simulink model "scara_host"  (Simulink 8.1)
settings: Solver=FixedStepDiscrete  StartTime=0.0  StopTime=inf  RelTol=1e-3
libraries: simulink x7
settings Model: Creator=Sr Antonio  LastModifiedBy=sp
settings DebuggingCC: FcnCallInpInsideContextMsg=EnableAllAsWarning

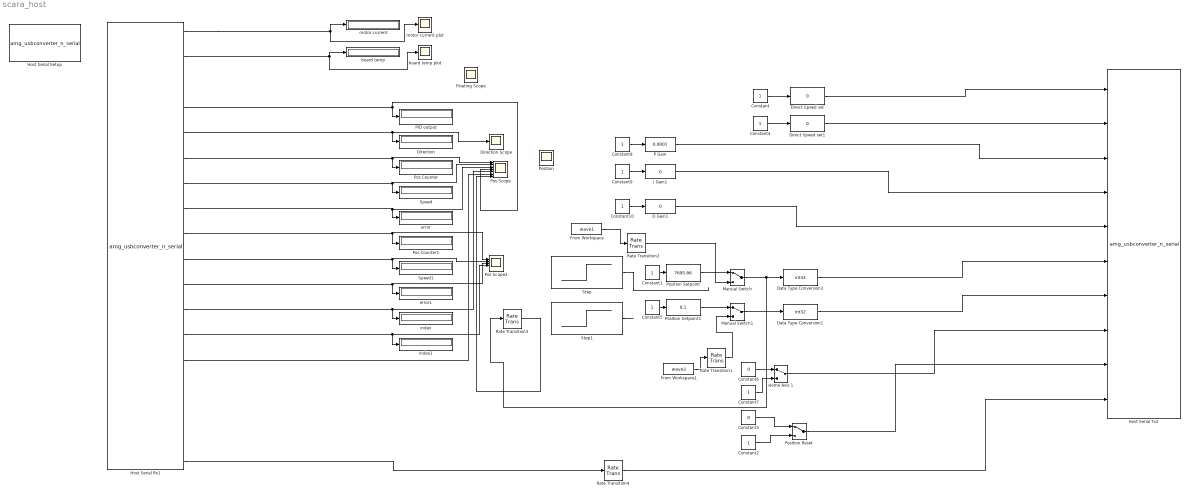
== system scara_host ==
  Constant{,4,8..10} (5 alike) : Constant
  Constant{1..2,5,7} (4 alike) : Constant  OutDataTypeStr=int32
  Constant3 : Constant  Value=0  OutDataTypeStr=int32
  Constant6 : Constant  Value=0  OutDataTypeStr=int32
  D Gain1 : simulink/Math Operations/Slider Gain  low=0  gain=0  high=10000
  Data Type Conversion1 : DataTypeConversion  OutDataTypeStr=int32
  Data Type Conversion3 : DataTypeConversion  OutDataTypeStr=int32
  Direct Speed set : simulink/Math Operations/Slider Gain  low=-1  gain=0  high=1
  Direct Speed set1 : simulink/Math Operations/Slider Gain  low=-1  gain=0  high=1
  Direction : Display
  Direction Scope : Scope
      settings: YMin=3e+07  YMax=3.35e+07  SaveName=ScopeData3
  Floating Scope : Scope
      settings: Floating=on  YMin=-12000  YMax=1000  SaveName=ScopeData5
  From Workspace : FromWorkspace  VariableName=wave1  SampleTime=0.001  Interpolate=off  OutputAfterFinalValue=Cyclic repetition
  From Workspace1 : FromWorkspace  VariableName=wave2  SampleTime=0.01  Interpolate=off  OutputAfterFinalValue=Cyclic repetition
  Home Axis 1 : ManualSwitch
  Host Serial Rx1 : S-Function  Priority=1  FunctionName=amg_usbconverter_n_serial  Parameters=configuration,port,transfer,baudrate,stopbit,inputtype,outputtype,binheaderarray,binterminatorarray,asciiheader,asciiterminator,bindatalength,packetmode,timeout,sampletime,sampletimestr,blockid  EnableBusSupport=off  mask(amg_usbconverter_n_serial){configuration=Rx, port=COM6, baudrate=115200, databits=8, parity=None, stopbit=1, flowcontrol=None, advanceoptions=off, rxbuffersize=2048, txbuffersize=2048, transfer=Blocking, timeout=2, packetmode=Binary, binheader='0E 0E', binterminator='0A 0A', porttype_double=4, porttype_single=0, porttype_int8=0, porttype_uint8=0, porttype_int16=0, porttype_uint16=0, porttype_int32=14, porttype_uint32=0, asciiformat='%d,%f', rx_asciiterminator=LF (0x0A - "\n"), tx_asciiterminator=LF (0x0A - "\n"), inputtype=[0], outputtype=[18  0 0 0 0 6 6 6 6 6 6 6 6 6 6 6 6 6 6], binheaderarray=[2 14  14], binterminatorarray=[2 10  10], bindatalength=88, asciiheader=['%d,%f' uint8(10)], asciiterminator=[1 10], sampletime=0.001, sampletimestr=, blockid=HostSerialRx1}
      mask prompts: baudrate "Baud rate (bps)"; databits "Data bits"; stopbit "Stop bit"; flowcontrol "Hardware flow control"; advanceoptions "Advance options"; rxbuffersize "Rx buffer size (bytes)"; txbuffersize "Tx buffer size (bytes)"; timeout "Wait time-out (Seconds)"; packetmode "Packet mode"; binheader "Binary header (example: '7E 7E')"; binterminator "Binary terminator (example: '03 03')"; porttype_double "Number of data port, type DOUBLE"; porttype_single "Number of data port, type SINGLE"; porttype_int8 "Number of data port, type INT8"; porttype_uint8 "Number of data port, type UINT8"; porttype_int16 "Number of data port, type INT16"; porttype_uint16 "Number of data port, type UINT16"; porttype_int32 "Number of data port, type INT32"; porttype_uint32 "Number of data port, type UINT32"; asciiformat "Ascii format"; rx_asciiterminator "End of packet"; tx_asciiterminator "End of packet"; inputtype "Input data type"; outputtype "Output data type"; binheaderarray "Binary header"; binterminatorarray "Binary terminator"; bindatalength "Binary data length"; asciiheader "Ascii header (printf format)"; asciiterminator "Ascii terminator"; sampletime "Sample time (sec)"; sampletimestr "Compiled sample time (sec) in string"
      mask init:
      | amg_usbconverter_n_serial_callback('init');
      mask Help: web(fullfile(waijungdocroot,'amg_usbconverter_n_uart.htm'), '-browser')
      mask TypeOptions configuration: Setup | Tx | Rx
      mask Callback configuration: amg_usbconverter_n_serial_callback('configuration');
      mask TypeOptions port: COM6
      mask Callback port: amg_usbconverter_n_serial_callback('port');
      mask Callback baudrate: amg_usbconverter_n_serial_callback('baudrate');
      mask TypeOptions databits: 8
      mask TypeOptions parity: None
      mask TypeOptions stopbit: 1 | 1.5 | 2
      mask TypeOptions flowcontrol: None | RTS | CTS | RTS/CTS
      mask Callback flowcontrol: amg_usbconverter_n_serial_callback('flowcontrol');
      mask Callback advanceoptions: amg_usbconverter_n_serial_callback('advanceoptions');
      mask TypeOptions rxbuffersize: 16 | 32 | 64 | 128 | 256 | 512 | 1024 | 2048
      mask TypeOptions txbuffersize: 16 | 32 | 64 | 128 | 256 | 512 | 1024 | 2048
      mask TypeOptions transfer: Blocking | Non-Blocking
      mask Callback transfer: amg_usbconverter_n_serial_callback('transfer');
      mask TypeOptions packetmode: Ascii | Binary
      mask Callback packetmode: amg_usbconverter_n_serial_callback('packetmode');
      mask Callback binheader: amg_usbconverter_n_serial_callback('binheader');
      mask Callback binterminator: amg_usbconverter_n_serial_callback('binterminator');
      mask Callback porttype_double: amg_usbconverter_n_serial_callback('porttype');
      mask Callback porttype_single: amg_usbconverter_n_serial_callback('porttype');
      mask Callback porttype_int8: amg_usbconverter_n_serial_callback('porttype');
      mask Callback porttype_uint8: amg_usbconverter_n_serial_callback('porttype');
      mask Callback porttype_int16: amg_usbconverter_n_serial_callback('porttype');
      mask Callback porttype_uint16: amg_usbconverter_n_serial_callback('porttype');
      mask Callback porttype_int32: amg_usbconverter_n_serial_callback('porttype');
      mask Callback porttype_uint32: amg_usbconverter_n_serial_callback('porttype');
      mask Callback asciiformat: amg_usbconverter_n_serial_callback('asciiformat');
      mask TypeOptions rx_asciiterminator: CR (0x0D - "\r") | LF (0x0A - "\n") | CRLF (0x0D 0x0A - "\r\n")
      mask Callback rx_asciiterminator: amg_usbconverter_n_serial_callback('rx_asciiterminator');
      mask TypeOptions tx_asciiterminator: CR (0x0D - "\r") | LF (0x0A - "\n") | CRLF (0x0D 0x0A - "\r\n") | None
      mask Callback tx_asciiterminator: amg_usbconverter_n_serial_callback('tx_asciiterminator');
      mask Callback sampletime: amg_usbconverter_n_serial_callback('sampletime');
      mask Callback sampletimestr: amg_usbconverter_n_serial_callback('sampletimestr');
      mask Callback blockid: amg_usbconverter_n_serial_callback('blockid');
      mask Display: text(0.05, 0.5, 'Obsolete !!!\nPort: COM6\nPacket: Binary\nTransfer: Blocking\nTs (sec): 0.001','ver','middle','hor','left');port_label('output', 1,'double');port_label('output', 2,'double');port_label('output', 3,'double');port_label('output', 4,'double');port_label('output', 5,'int32');port_label('output', 6,'int32');port_label('output', 7,'int32');port_label('output', 8,'int32');port_label('output', 9,'int32');port_label('output', 10,'int32');port_label('output', 11,'int32');port_label('output', 12,'int32');port_label('output', 13,'int32');port_label('output', 14,'int32');port_label('output', 15,'int32');port_label('output', 16,'int32');port_label('output', 17,'int32');port_label('output', 18,'int32');
  Host Serial Setup : S-Function  Priority=1  FunctionName=amg_usbconverter_n_serial  Parameters=configuration,port,transfer,baudrate,stopbit,inputtype,outputtype,binheaderarray,binterminatorarray,asciiheader,asciiterminator,bindatalength,packetmode,timeout,sampletime,sampletimestr,blockid  EnableBusSupport=off  mask(amg_usbconverter_n_serial){configuration=Setup, port=COM6, baudrate=10000000, databits=8, parity=None, stopbit=1, flowcontrol=None, advanceoptions=off, rxbuffersize=2048, txbuffersize=2048, transfer=Blocking, timeout=5, packetmode=Binary, binheader='7E 7E', binterminator='03 03', porttype_double=1, porttype_single=0, porttype_int8=1, porttype_uint8=0, porttype_int16=0, porttype_uint16=0, porttype_int32=0, porttype_uint32=0, asciiformat='%d,%f', rx_asciiterminator=CRLF (0x0D 0x0A - "\r\n"), tx_asciiterminator=CR (0x0D - "\r"), inputtype=[0], outputtype=[0], binheaderarray=[2 126  126], binterminatorarray=[2 3  3], bindatalength=0, asciiheader='', asciiterminator=[0], sampletime=inf, sampletimestr=, blockid=HostSerialSetup}
      mask prompts: baudrate "Baud rate (bps)"; databits "Data bits"; stopbit "Stop bit"; flowcontrol "Hardware flow control"; advanceoptions "Advance options"; rxbuffersize "Rx buffer size (bytes)"; txbuffersize "Tx buffer size (bytes)"; timeout "Wait time-out (Seconds)"; packetmode "Packet mode"; binheader "Binary header (example: '7E 7E')"; binterminator "Binary terminator (example: '03 03')"; porttype_double "Number of data port, type DOUBLE"; porttype_single "Number of data port, type SINGLE"; porttype_int8 "Number of data port, type INT8"; porttype_uint8 "Number of data port, type UINT8"; porttype_int16 "Number of data port, type INT16"; porttype_uint16 "Number of data port, type UINT16"; porttype_int32 "Number of data port, type INT32"; porttype_uint32 "Number of data port, type UINT32"; asciiformat "Ascii format"; rx_asciiterminator "End of packet"; tx_asciiterminator "End of packet"; inputtype "Input data type"; outputtype "Output data type"; binheaderarray "Binary header"; binterminatorarray "Binary terminator"; bindatalength "Binary data length"; asciiheader "Ascii header (printf format)"; asciiterminator "Ascii terminator"; sampletime "Sample time (sec)"; sampletimestr "Compiled sample time (sec) in string"
      mask init:
      | amg_usbconverter_n_serial_callback('init');
      mask Help: web(fullfile(waijungdocroot,'amg_usbconverter_n_uart.htm'), '-browser')
      mask TypeOptions configuration: Setup | Tx | Rx
      mask Callback configuration: amg_usbconverter_n_serial_callback('configuration');
      mask TypeOptions port: COM6
      mask Callback port: amg_usbconverter_n_serial_callback('port');
      mask Callback baudrate: amg_usbconverter_n_serial_callback('baudrate');
      mask TypeOptions databits: 8
      mask TypeOptions parity: None
      mask TypeOptions stopbit: 1 | 1.5 | 2
      mask TypeOptions flowcontrol: None | RTS | CTS | RTS/CTS
      mask Callback flowcontrol: amg_usbconverter_n_serial_callback('flowcontrol');
      mask Callback advanceoptions: amg_usbconverter_n_serial_callback('advanceoptions');
      mask TypeOptions rxbuffersize: 16 | 32 | 64 | 128 | 256 | 512 | 1024 | 2048
      mask TypeOptions txbuffersize: 16 | 32 | 64 | 128 | 256 | 512 | 1024 | 2048
      mask TypeOptions transfer: Blocking | Non-Blocking
      mask Callback transfer: amg_usbconverter_n_serial_callback('transfer');
      mask TypeOptions packetmode: Ascii | Binary
      mask Callback packetmode: amg_usbconverter_n_serial_callback('packetmode');
      mask Callback binheader: amg_usbconverter_n_serial_callback('binheader');
      mask Callback binterminator: amg_usbconverter_n_serial_callback('binterminator');
      mask Callback porttype_double: amg_usbconverter_n_serial_callback('porttype');
      mask Callback porttype_single: amg_usbconverter_n_serial_callback('porttype');
      mask Callback porttype_int8: amg_usbconverter_n_serial_callback('porttype');
      mask Callback porttype_uint8: amg_usbconverter_n_serial_callback('porttype');
      mask Callback porttype_int16: amg_usbconverter_n_serial_callback('porttype');
      mask Callback porttype_uint16: amg_usbconverter_n_serial_callback('porttype');
      mask Callback porttype_int32: amg_usbconverter_n_serial_callback('porttype');
      mask Callback porttype_uint32: amg_usbconverter_n_serial_callback('porttype');
      mask Callback asciiformat: amg_usbconverter_n_serial_callback('asciiformat');
      mask TypeOptions rx_asciiterminator: CR (0x0D - "\r") | LF (0x0A - "\n") | CRLF (0x0D 0x0A - "\r\n")
      mask Callback rx_asciiterminator: amg_usbconverter_n_serial_callback('rx_asciiterminator');
      mask TypeOptions tx_asciiterminator: CR (0x0D - "\r") | LF (0x0A - "\n") | CRLF (0x0D 0x0A - "\r\n") | None
      mask Callback tx_asciiterminator: amg_usbconverter_n_serial_callback('tx_asciiterminator');
      mask Callback sampletime: amg_usbconverter_n_serial_callback('sampletime');
      mask Callback sampletimestr: amg_usbconverter_n_serial_callback('sampletimestr');
      mask Callback blockid: amg_usbconverter_n_serial_callback('blockid');
      mask Display: text(0.5, 0.5, 'Port: COM6\nBaud (Bps): 10000000\nFrame: 8-None-1','ver','middle','hor','center');
  Host Serial Tx2 : S-Function  Priority=1  FunctionName=amg_usbconverter_n_serial  Parameters=configuration,port,transfer,baudrate,stopbit,inputtype,outputtype,binheaderarray,binterminatorarray,asciiheader,asciiterminator,bindatalength,packetmode,timeout,sampletime,sampletimestr,blockid  EnableBusSupport=off  mask(amg_usbconverter_n_serial){configuration=Tx, port=COM6, baudrate=115200, databits=8, parity=None, stopbit=1, flowcontrol=None, advanceoptions=off, rxbuffersize=2048, txbuffersize=2048, transfer=Blocking, timeout=2, packetmode=Binary, binheader='7E 7E', binterminator='03 03', porttype_double=5, porttype_single=0, porttype_int8=0, porttype_uint8=0, porttype_int16=0, porttype_uint16=0, porttype_int32=5, porttype_uint32=0, asciiformat='%d,%f', rx_asciiterminator=CRLF (0x0D 0x0A - "\r\n"), tx_asciiterminator=LF (0x0A - "\n"), inputtype=[10  0 0 0 0 0 6 6 6 6 6], outputtype=[0], binheaderarray=[2 126  126], binterminatorarray=[2 3  3], bindatalength=60, asciiheader=['%d,%f' uint8(10)], asciiterminator=[1 10], sampletime=0.001, sampletimestr=, blockid=HostSerialTx2}
      mask prompts: baudrate "Baud rate (bps)"; databits "Data bits"; stopbit "Stop bit"; flowcontrol "Hardware flow control"; advanceoptions "Advance options"; rxbuffersize "Rx buffer size (bytes)"; txbuffersize "Tx buffer size (bytes)"; timeout "Wait time-out (Seconds)"; packetmode "Packet mode"; binheader "Binary header (example: '7E 7E')"; binterminator "Binary terminator (example: '03 03')"; porttype_double "Number of data port, type DOUBLE"; porttype_single "Number of data port, type SINGLE"; porttype_int8 "Number of data port, type INT8"; porttype_uint8 "Number of data port, type UINT8"; porttype_int16 "Number of data port, type INT16"; porttype_uint16 "Number of data port, type UINT16"; porttype_int32 "Number of data port, type INT32"; porttype_uint32 "Number of data port, type UINT32"; asciiformat "Ascii format"; rx_asciiterminator "End of packet"; tx_asciiterminator "End of packet"; inputtype "Input data type"; outputtype "Output data type"; binheaderarray "Binary header"; binterminatorarray "Binary terminator"; bindatalength "Binary data length"; asciiheader "Ascii header (printf format)"; asciiterminator "Ascii terminator"; sampletime "Sample time (sec)"; sampletimestr "Compiled sample time (sec) in string"
      mask init:
      | amg_usbconverter_n_serial_callback('init');
      mask Help: web(fullfile(waijungdocroot,'amg_usbconverter_n_uart.htm'), '-browser')
      mask TypeOptions configuration: Setup | Tx | Rx
      mask Callback configuration: amg_usbconverter_n_serial_callback('configuration');
      mask TypeOptions port: COM6
      mask Callback port: amg_usbconverter_n_serial_callback('port');
      mask Callback baudrate: amg_usbconverter_n_serial_callback('baudrate');
      mask TypeOptions databits: 8
      mask TypeOptions parity: None
      mask TypeOptions stopbit: 1 | 1.5 | 2
      mask TypeOptions flowcontrol: None | RTS | CTS | RTS/CTS
      mask Callback flowcontrol: amg_usbconverter_n_serial_callback('flowcontrol');
      mask Callback advanceoptions: amg_usbconverter_n_serial_callback('advanceoptions');
      mask TypeOptions rxbuffersize: 16 | 32 | 64 | 128 | 256 | 512 | 1024 | 2048
      mask TypeOptions txbuffersize: 16 | 32 | 64 | 128 | 256 | 512 | 1024 | 2048
      mask TypeOptions transfer: Blocking | Non-Blocking
      mask Callback transfer: amg_usbconverter_n_serial_callback('transfer');
      mask TypeOptions packetmode: Ascii | Binary
      mask Callback packetmode: amg_usbconverter_n_serial_callback('packetmode');
      mask Callback binheader: amg_usbconverter_n_serial_callback('binheader');
      mask Callback binterminator: amg_usbconverter_n_serial_callback('binterminator');
      mask Callback porttype_double: amg_usbconverter_n_serial_callback('porttype');
      mask Callback porttype_single: amg_usbconverter_n_serial_callback('porttype');
      mask Callback porttype_int8: amg_usbconverter_n_serial_callback('porttype');
      mask Callback porttype_uint8: amg_usbconverter_n_serial_callback('porttype');
      mask Callback porttype_int16: amg_usbconverter_n_serial_callback('porttype');
      mask Callback porttype_uint16: amg_usbconverter_n_serial_callback('porttype');
      mask Callback porttype_int32: amg_usbconverter_n_serial_callback('porttype');
      mask Callback porttype_uint32: amg_usbconverter_n_serial_callback('porttype');
      mask Callback asciiformat: amg_usbconverter_n_serial_callback('asciiformat');
      mask TypeOptions rx_asciiterminator: CR (0x0D - "\r") | LF (0x0A - "\n") | CRLF (0x0D 0x0A - "\r\n")
      mask Callback rx_asciiterminator: amg_usbconverter_n_serial_callback('rx_asciiterminator');
      mask TypeOptions tx_asciiterminator: CR (0x0D - "\r") | LF (0x0A - "\n") | CRLF (0x0D 0x0A - "\r\n") | None
      mask Callback tx_asciiterminator: amg_usbconverter_n_serial_callback('tx_asciiterminator');
      mask Callback sampletime: amg_usbconverter_n_serial_callback('sampletime');
      mask Callback sampletimestr: amg_usbconverter_n_serial_callback('sampletimestr');
      mask Callback blockid: amg_usbconverter_n_serial_callback('blockid');
      mask Display: text(0.95, 0.5, 'Port: COM6\nPacket: Binary\nTransfer: Blocking\nTs (sec): 0.001','ver','middle','hor','right');port_label('input', 1,'double');port_label('input', 2,'double');port_label('input', 3,'double');port_label('input', 4,'double');port_label('input', 5,'double');port_label('input', 6,'int32');port_label('input', 7,'int32');port_label('input', 8,'int32');port_label('input', 9,'int32');port_label('input', 10,'int32');
  I Gain1 : simulink/Math Operations/Slider Gain  low=0  gain=0  high=0.1
  Manual Switch : ManualSwitch
  Manual Switch1 : ManualSwitch
  P Gain : simulink/Math Operations/Slider Gain  low=1e-05  gain=0.0001  high=1
  PID output : Display
  Pos Counter : Display
      settings: Format=bank
  Pos Counter1 : Display
      settings: Format=bank
  Pos Scope : Scope  NumInputPorts=7
      settings: ShowLegends=on  YMin=2500~-70~-5000~-1~-200~-5~-17500  YMax=22500~80~5000~1~200~5~0
  Pos Scope2 : Scope  NumInputPorts=5
      settings: ShowLegends=on  YMin=16000~-25~-5000~0~-5  YMax=27000~25~6000~5~5
  Position : Scope
      settings: Floating=on  TimeRange=20  YMin=-10000  YMax=22500  SaveName=ScopeData2
  Position Reset : ManualSwitch
  Position Setpoint : simulink/Math Operations/Slider Gain  low=-10000  gain=7695.86  high=10000
  Position Setpoint1 : simulink/Math Operations/Slider Gain  low=-10000  gain=0.1  high=10000
  Rate Transition1 : RateTransition  OutPortSampleTimeOpt=Inherit  OutPortSampleTime=0.001
  Rate Transition2 : RateTransition  OutPortSampleTimeOpt=Inherit  OutPortSampleTime=0.001
  Rate Transition3 : RateTransition  Integrity=off  OutPortSampleTimeOpt=Inherit  OutPortSampleTime=0.001
  Rate Transition4 : RateTransition  OutPortSampleTimeOpt=Inherit  OutPortSampleTime=0.001
  Speed : Display
  Speed1 : Display
  Step : Step  After=10000  SampleTime=0.001
  Step1 : Step  After=1000  SampleTime=0.001
  board temp : Display
      settings: Format=bank
  board temp plot : Scope
      settings: TimeRange=5  YMin=0  YMax=4000  SaveName=ScopeData9  SampleTime=0.01
  error : Display
      settings: Format=bank
  error1 : Display
      settings: Format=bank
  index : Display
      settings: Format=bank
  index1 : Display
      settings: Format=bank
  motor current : Display
      settings: Format=bank
  motor current plot : Scope
      settings: TimeRange=5  YMin=0  YMax=4000  SaveName=ScopeData4  SampleTime=0.01
  wires:
  Host Serial Rx1/5 -> Direction/1, Direction Scope/1
  Host Serial Rx1/7 -> Speed/1, Pos Scope/2
  Host Serial Rx1/6 -> Pos Counter/1, Pos Scope/1
  Host Serial Rx1/8 -> error/1, Pos Scope/3
  Host Serial Rx1/4 -> PID output/1, Pos Scope/4
  Direct Speed set/1 -> Host Serial Tx2/1
  Constant/1 -> Direct Speed set/1
  Constant1/1 -> Position Setpoint/1
  Manual Switch/1 -> Rate Transition3/1, Data Type Conversion3/1
  Step/1 -> ?
  Position Reset/1 -> Host Serial Tx2/9
  Constant2/1 -> Position Reset/2
  Constant3/1 -> Position Reset/1
  Data Type Conversion3/1 -> Host Serial Tx2/6
  Position Setpoint/1 -> Manual Switch/1
  Direct Speed set1/1 -> Host Serial Tx2/2
  Constant4/1 -> Direct Speed set1/1
  Constant5/1 -> Position Setpoint1/1
  Manual Switch1/1 -> Data Type Conversion1/1
  Step1/1 -> ?
  Position Setpoint1/1 -> Manual Switch1/1
  Data Type Conversion1/1 -> Host Serial Tx2/7
  Host Serial Rx1/10 -> Speed1/1, Pos Scope2/2
  Host Serial Rx1/9 -> Pos Counter1/1, Pos Scope2/1
  Host Serial Rx1/11 -> error1/1, Pos Scope2/3
  Host Serial Rx1/2 -> board temp plot/1, board temp/1
  Home Axis 1/1 -> Host Serial Tx2/8
  Host Serial Rx1/12 -> index/1, Pos Scope/5
  Host Serial Rx1/13 -> index1/1, Pos Scope2/4
  Constant6/1 -> Home Axis 1/1
  Constant7/1 -> Home Axis 1/2
  Host Serial Rx1/14 -> Pos Scope/6
  From Workspace/1 -> Rate Transition2/1
  From Workspace1/1 -> Rate Transition1/1
  Rate Transition1/1 -> Manual Switch1/2
  Rate Transition2/1 -> Manual Switch/2
  Rate Transition3/1 -> Pos Scope/7
  Host Serial Rx1/18 -> Rate Transition4/1
  Rate Transition4/1 -> Host Serial Tx2/10
  Constant8/1 -> P Gain/1
  P Gain/1 -> Host Serial Tx2/3
  Constant9/1 -> I Gain1/1
  I Gain1/1 -> Host Serial Tx2/4
  Constant10/1 -> D Gain1/1
  D Gain1/1 -> Host Serial Tx2/5
  Host Serial Rx1/1 -> motor current plot/1, motor current/1
